simulink model "EMB_Lost_full"  (R2022a)
settings: Solver=VariableStepAuto  StartTime=0.0  StopTime=2  RelTol=1e-3
libraries: slpidlib x24, spsDCVoltageSourceLib x4, spsPermanentMagnetSynchronousMachineLib x4, spsSVPWMGenerator2LevelLib x4, spsUniversalBridgeLib x4, spsdq0toAlphaBetaZeroLib x4, spspowerguiLib x4
(part 3 of 3)

== system EMB_Lost_full/EMB_Frr/Ud_PI ==
  Ud_Target : Inport
  Ud_Actual : Inport  Port=2
  PID Controller : slpidlib/PID Controller  Controller=PI  Form=Parallel  TimeDomain=Continuous-time  UseExternalTs=off  SampleTime=-1  IntegratorMethod=Forward Euler  FilterMethod=Forward Euler  ControllerParametersSource=internal  P=0.12  I=0  UseKiTs=off  D=0.01  N=5  UseFilter=on  TunerSelectOption=Transfer Function Based (PID Tuner App)  InitialConditionSource=internal  InitialConditionForIntegrator=0  InitialConditionForFilter=0  DifferentiatorICPrevScaledInput=0  ExternalReset=none  TrackingMode=off  Kt=1  LimitOutput=on  SatLimitsSource=internal  UpperSaturationLimit=24  LowerSaturationLimit=-24  LinearizeAsGain=on  AntiWindupMode=none  Kb=1  POutMin=[]  POutMax=[]  IOutMin=[]  IOutMax=[]  DOutMin=[]  DOutMax=[]  NOutMin=[]  NOutMax=[]  SumOutMin=[]  SumOutMax=[]  SaturationOutMin=[]  SaturationOutMax=[]  PParamMin=[]  PParamMax=[]  IParamMin=[]  IParamMax=[]  DParamMin=[]  DParamMax=[]  NParamMin=[]  NParamMax=[]  KbParamMin=[]  KbParamMax=[]  KtParamMin=[]  KtParamMax=[]  KbOutMin=[]  KbOutMax=[]  KtOutMin=[]  KtOutMax=[]  IntegratorOutMin=[]  IntegratorOutMax=[]  FilterOutMin=[]  FilterOutMax=[]  SumI1OutMin=[]  SumI1OutMax=[]  SumI2OutMin=[]  SumI2OutMax=[]  SumI3OutMin=[]  SumI3OutMax=[]  SumI4OutMin=[]  SumI4OutMax=[]  SumDOutMin=[]  SumDOutMax=[]  DifferentiatorOutMin=[]  DifferentiatorOutMax=[]  FilterDiffOutCoefMin=[]  FilterDiffOutCoefMax=[]  ReciprocalOutMin=[]  ReciprocalOutMax=[]  SumDenOutMin=[]  SumDenOutMax=[]  SumNumOutMin=[]  SumNumOutMax=[]  DivideOutMin=[]  DivideOutMax=[]  UdiffTsProdOutMin=[]  UdiffTsProdOutMax=[]  NTsProdOutMin=[]  NTsProdOutMax=[]  UintegralTsProdOutMin=[]  UintegralTsProdOutMax=[]  UngainTsProdOutMin=[]  UngainTsProdOutMax=[]  IntegratorContinuousStateAttributes=''  IntegratorStateMustResolveToSignalObject=off  IntegratorRTWStateStorageClass=Auto  FilterContinuousStateAttributes=''  FilterStateMustResolveToSignalObject=off  FilterRTWStateStorageClass=Auto  ParallelPVariant=InternalParameters  IdealPVariant=Disabled  IVariant=InternalParameters  DVariant=Disabled  IntegratorVariant=Continuous  SatVariant=Enabled  AWVariant=Passthrough  PCopyVariant=Disabled  TRVariant=Disabled  FdbkBlocksVariant=Forward  IdealPFdbkVariant=Disabled  SatFdbkVariant=Disabled  DerivativeFilterVariant=Disabled  NVariant=Disabled  NCopyVariant=Disabled_SignalSpec  FilterICVariant=Disabled  IntegratorICVariant=InternalICs  ExternalResetVariant=Disabled  TRSumVariant=Passthrough  SumFdbkVariant=Disabled  SumVariant=Sum_PI  TsampFilterVariant=InternalTs  TsampNgainVariant=Passthrough  TsampIntegralVariant=Passthrough  ExternalSaturationOutDataTypeStr=Inherit: Same as second input  aMode=0
  Sum : Sum  Inputs=|+-
  Ud : Outport
  wires:
  Sum/1 -> PID Controller/1
  Ud_Actual/1 -> Sum/2
  Ud_Target/1 -> Sum/1
  PID Controller/1 -> Ud/1

== system EMB_Lost_full/EMB_Frr/Uq_PI ==
  Uq_Target : Inport
  Uq_Actual : Inport  Port=2
  PID Controller : slpidlib/PID Controller  Controller=PI  Form=Parallel  TimeDomain=Continuous-time  UseExternalTs=off  SampleTime=-1  IntegratorMethod=Forward Euler  FilterMethod=Forward Euler  ControllerParametersSource=internal  P=0.12  I=0  UseKiTs=off  D=0.01  N=5  UseFilter=on  TunerSelectOption=Transfer Function Based (PID Tuner App)  InitialConditionSource=internal  InitialConditionForIntegrator=0  InitialConditionForFilter=0  DifferentiatorICPrevScaledInput=0  ExternalReset=none  TrackingMode=off  Kt=1  LimitOutput=on  SatLimitsSource=internal  UpperSaturationLimit=24  LowerSaturationLimit=-24  LinearizeAsGain=on  AntiWindupMode=none  Kb=1  POutMin=[]  POutMax=[]  IOutMin=[]  IOutMax=[]  DOutMin=[]  DOutMax=[]  NOutMin=[]  NOutMax=[]  SumOutMin=[]  SumOutMax=[]  SaturationOutMin=[]  SaturationOutMax=[]  PParamMin=[]  PParamMax=[]  IParamMin=[]  IParamMax=[]  DParamMin=[]  DParamMax=[]  NParamMin=[]  NParamMax=[]  KbParamMin=[]  KbParamMax=[]  KtParamMin=[]  KtParamMax=[]  KbOutMin=[]  KbOutMax=[]  KtOutMin=[]  KtOutMax=[]  IntegratorOutMin=[]  IntegratorOutMax=[]  FilterOutMin=[]  FilterOutMax=[]  SumI1OutMin=[]  SumI1OutMax=[]  SumI2OutMin=[]  SumI2OutMax=[]  SumI3OutMin=[]  SumI3OutMax=[]  SumI4OutMin=[]  SumI4OutMax=[]  SumDOutMin=[]  SumDOutMax=[]  DifferentiatorOutMin=[]  DifferentiatorOutMax=[]  FilterDiffOutCoefMin=[]  FilterDiffOutCoefMax=[]  ReciprocalOutMin=[]  ReciprocalOutMax=[]  SumDenOutMin=[]  SumDenOutMax=[]  SumNumOutMin=[]  SumNumOutMax=[]  DivideOutMin=[]  DivideOutMax=[]  UdiffTsProdOutMin=[]  UdiffTsProdOutMax=[]  NTsProdOutMin=[]  NTsProdOutMax=[]  UintegralTsProdOutMin=[]  UintegralTsProdOutMax=[]  UngainTsProdOutMin=[]  UngainTsProdOutMax=[]  IntegratorContinuousStateAttributes=''  IntegratorStateMustResolveToSignalObject=off  IntegratorRTWStateStorageClass=Auto  FilterContinuousStateAttributes=''  FilterStateMustResolveToSignalObject=off  FilterRTWStateStorageClass=Auto  ParallelPVariant=InternalParameters  IdealPVariant=Disabled  IVariant=InternalParameters  DVariant=Disabled  IntegratorVariant=Continuous  SatVariant=Enabled  AWVariant=Passthrough  PCopyVariant=Disabled  TRVariant=Disabled  FdbkBlocksVariant=Forward  IdealPFdbkVariant=Disabled  SatFdbkVariant=Disabled  DerivativeFilterVariant=Disabled  NVariant=Disabled  NCopyVariant=Disabled_SignalSpec  FilterICVariant=Disabled  IntegratorICVariant=InternalICs  ExternalResetVariant=Disabled  TRSumVariant=Passthrough  SumFdbkVariant=Disabled  SumVariant=Sum_PI  TsampFilterVariant=InternalTs  TsampNgainVariant=Passthrough  TsampIntegralVariant=Passthrough  ExternalSaturationOutDataTypeStr=Inherit: Same as second input  aMode=0
  Sum : Sum  Inputs=|+-
  Uq : Outport
  wires:
  Sum/1 -> PID Controller/1
  Uq_Actual/1 -> Sum/2
  PID Controller/1 -> Uq/1
  Uq_Target/1 -> Sum/1

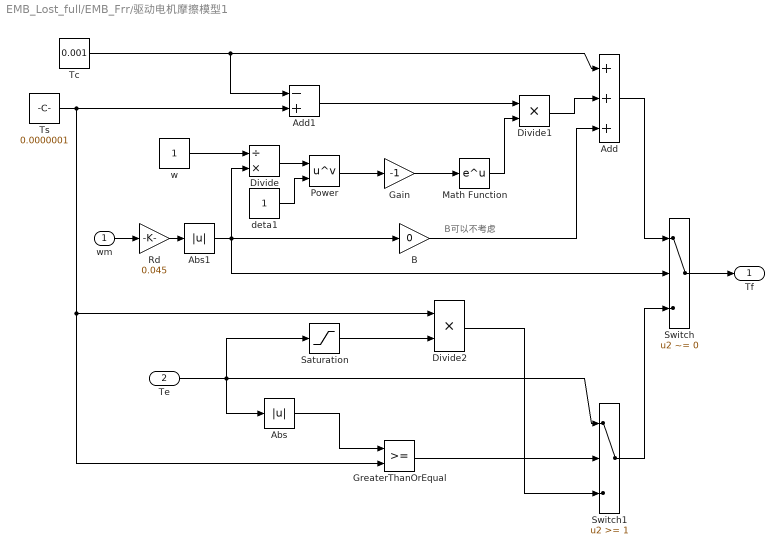
== system EMB_Lost_full/EMB_Frr/驱动电机摩擦模型1 ==
  note: B可以不考虑
  wm : Inport
  Te : Inport  Port=2
  Abs : Abs  SaturateOnIntegerOverflow=off
  Abs1 : Abs  SaturateOnIntegerOverflow=off
  Add : Sum  Inputs=+++
  Add1 : Sum  Inputs=-+
  B : Gain  Gain=0
  Divide : Product  Inputs=/*
  Divide1 : Product  Inputs=**
  Divide2 : Product  Inputs=**
  Gain : Gain  Gain=-1
  GreaterThanOrEqual : RelationalOperator  OutDataTypeStr=boolean  RndMeth=Simplest  InputSameDT=off
  Math Function : Math
  Power : Math  Operator=pow
  Rd : Gain  Gain=0.045
  Saturation : Saturate  UpperLimit=1  LowerLimit=-1
  Switch : Switch  Criteria=u2 ~= 0  SaturateOnIntegerOverflow=off  InputSameDT=off
  Switch1 : Switch  Threshold=1  SaturateOnIntegerOverflow=off  InputSameDT=off
  Tc : Constant  Value=0.001
  Ts : Constant  Value=0.0000001
  deta1 : Constant
  w : Constant
  Tf : Outport
  wires:
  Tc/1 -> Add1/1, Add/1
  Ts/1 -> Add1/2, Divide2/1, GreaterThanOrEqual/2
  B/1 -> Add/3
  w/1 -> Divide/1
  Divide/1 -> Power/1
  deta1/1 -> Power/2
  Add1/1 -> Divide1/1
  Math Function/1 -> Divide1/2
  Divide1/1 -> Add/2
  Power/1 -> Gain/1
  Gain/1 -> Math Function/1
  Switch/1 -> Tf/1
  Add/1 -> Switch/1
  Switch1/1 -> Switch/3
  Te/1 -> Saturation/1, Switch1/1, Abs/1
  Abs/1 -> GreaterThanOrEqual/1
  GreaterThanOrEqual/1 -> Switch1/2
  Saturation/1 -> Divide2/2
  Divide2/1 -> Switch1/3
  wm/1 -> Rd/1
  Rd/1 -> Abs1/1
  Abs1/1 -> Switch/2, B/1, Divide/2

== matlab function EMB_Lost_full/EMB_Ffr/EMB执行机构1/MATLAB Function ==
  data: u input; FN output; TL output
function [FN,TL] = fcn(u)
L=5; %滚动丝杠导程，mm
ip=16;%行星齿轮减速器减速比
eta_s=0.92;%滚动丝杠传动效率
eta_p=0.96; %行星齿轮传动器传动效率
s=u-0.25;
Fn=0;

if s>0.3
    Fn = -1917.2*s^3+29010.8*s^2-10197.1*s+572.4;
    if Fn<53.12
        Fn=53.12;
    end
end
if s>0 && s<=0.3
    Fn = 295.1*s;
end
if s<0
    Fn = 0;
end
if Fn>=30000
    Fn=30000;
end
Tl = 0.001*Fn/((2*pi/L)*ip*eta_s*eta_p);
FN=Fn;
TL=Tl;

== matlab function EMB_Lost_full/EMB_Ffl/EMB执行机构1/MATLAB Function ==
  data: u input; FN output; TL output
function [FN,TL] = fcn(u)
L=5; %滚动丝杠导程，mm
ip=16;%行星齿轮减速器减速比
eta_s=0.92;%滚动丝杠传动效率
eta_p=0.96; %行星齿轮传动器传动效率
s=u-0.25;
Fn=0;

if s>0.3
    Fn = -1917.2*s^3+29010.8*s^2-10197.1*s+572.4;
    if Fn<53.12
        Fn=53.12;
    end
end
if s>0 && s<=0.3
    Fn = 295.1*s;
end
if s<0
    Fn = 0;
end
if Fn>=30000
    Fn=30000;
end
Tl = 0.001*Fn/((2*pi/L)*ip*eta_s*eta_p);
FN=Fn;
TL=Tl;

== matlab function EMB_Lost_full/EMB_Ffr/EMB执行策略判断2/MATLAB Function ==
  data: Fn_Target input; y output; Fn_Actual input; Fn_Threshold input
function y = fcn(Fn_Target,Fn_Actual,Fn_Threshold)
sign=0;

if Fn_Target>0 && Fn_Actual<Fn_Threshold
    sign=2;
end

if Fn_Target>=0 && Fn_Actual>Fn_Threshold
    sign=1;
end

if Fn_Target==0 && Fn_Actual<Fn_Threshold
    sign=3;
end
y=sign;

== matlab function EMB_Lost_full/EMB_Ffl/EMB执行策略判断2/MATLAB Function ==
  data: Fn_Target input; y output; Fn_Actual input; Fn_Threshold input
function y = fcn(Fn_Target,Fn_Actual,Fn_Threshold)
sign=0;

if Fn_Target>0 && Fn_Actual<Fn_Threshold
    sign=2;
end

if Fn_Target>=0 && Fn_Actual>Fn_Threshold
    sign=1;
end

if Fn_Target==0 && Fn_Actual<Fn_Threshold
    sign=3;
end
y=sign;

== matlab function EMB_Lost_full/EMB_Frl/EMB执行机构1/MATLAB Function ==
  data: u input; FN output; TL output
function [FN,TL] = fcn(u)
L=5; %滚动丝杠导程，mm
ip=16;%行星齿轮减速器减速比
eta_s=0.92;%滚动丝杠传动效率
eta_p=0.96; %行星齿轮传动器传动效率
s=u-0.25;
Fn=0;

if s>0.3
    Fn = -1917.2*s^3+29010.8*s^2-10197.1*s+572.4;
    if Fn<53.12
        Fn=53.12;
    end
end
if s>0 && s<=0.3
    Fn = 295.1*s;
end
if s<0
    Fn = 0;
end
if Fn>=30000
    Fn=30000;
end
Tl = 0.001*Fn/((2*pi/L)*ip*eta_s*eta_p);
FN=Fn;
TL=Tl;

== matlab function EMB_Lost_full/EMB_Frl/EMB执行策略判断2/MATLAB Function ==
  data: Fn_Target input; y output; Fn_Actual input; Fn_Threshold input
function y = fcn(Fn_Target,Fn_Actual,Fn_Threshold)
sign=0;

if Fn_Target>0 && Fn_Actual<Fn_Threshold
    sign=2;
end

if Fn_Target>=0 && Fn_Actual>Fn_Threshold
    sign=1;
end

if Fn_Target==0 && Fn_Actual<Fn_Threshold
    sign=3;
end
y=sign;

== matlab function EMB_Lost_full/EMB_Frr/EMB执行机构1/MATLAB Function ==
  data: u input; FN output; TL output
function [FN,TL] = fcn(u)
L=5; %滚动丝杠导程，mm
ip=16;%行星齿轮减速器减速比
eta_s=0.92;%滚动丝杠传动效率
eta_p=0.96; %行星齿轮传动器传动效率
s=u-0.25;
Fn=0;

if s>0.3
    Fn = -1917.2*s^3+29010.8*s^2-10197.1*s+572.4;
    if Fn<53.12
        Fn=53.12;
    end
end
if s>0 && s<=0.3
    Fn = 295.1*s;
end
if s<0
    Fn = 0;
end
if Fn>=30000
    Fn=30000;
end
Tl = 0.001*Fn/((2*pi/L)*ip*eta_s*eta_p);
FN=Fn;
TL=Tl;

== matlab function EMB_Lost_full/EMB_Frr/EMB执行策略判断2/MATLAB Function ==
  data: Fn_Target input; y output; Fn_Actual input; Fn_Threshold input
function y = fcn(Fn_Target,Fn_Actual,Fn_Threshold)
sign=0;

if Fn_Target>0 && Fn_Actual<Fn_Threshold
    sign=2;
end

if Fn_Target>=0 && Fn_Actual>Fn_Threshold
    sign=1;
end

if Fn_Target==0 && Fn_Actual<Fn_Threshold
    sign=3;
end
y=sign;

== matlab function EMB_Lost_full/EMB_Self-inspection/MATLAB Function ==
  data: Total_Fn input; Fn_Target output; lost input
function Fn_Target  = fcn(Total_Fn,lost)
m=1820;
g=9.8;
a=1.27;
b=1.42;
h=0.55;
Fnmax=6500;
Zx=Total_Fn/(m*g);
Beta_fr=(b+Zx*h)/(a-Zx*h);

Ffl_Target=0.5*Zx*m*g*Beta_fr/(1+Beta_fr);
Ffr_Target=Ffl_Target;
Frl_Target=0.5*Zx*m*g*(1-Beta_fr/(1+Beta_fr));
Frr_Target=Frl_Target;
if Ffr_Target>=Fnmax || Ffl_Target>=Fnmax
    Ffr_Target=Fnmax;
    Ffl_Target=Fnmax;
    Frl_Target=0.5*(Total_Fn-2*Fnmax);
    Frr_Target=0.5*(Total_Fn-2*Fnmax);
end
Fn_Target=[Ffl_Target,Ffr_Target,Frl_Target,Frr_Target];

if lost>=1
    switch lost
        case 1
        if Fn_Target(1)+Fn_Target(3)<=Fnmax
            Fn_Target(3)=Fn_Target(1)+Fn_Target(3);
        end
        if Fn_Target(1)+Fn_Target(3)>Fnmax && Total_Fn-Fn_Target(4)<=2*Fnmax
            Fn_Target(3)=Fnmax;
            Fn_Target(2)=Total_Fn-Fn_Target(4)-Fnmax;
        end
        if Total_Fn-Fn_Target(4)>2*Fnmax && Total_Fn<=3*Fnmax
            Fn_Target(3)=Fnmax;
            Fn_Target(2)=Fnmax;
            Fn_Target(4)=Total_Fn-2*Fnmax;
        end
        if Total_Fn>3*Fnmax
            Fn_Target(2)=Fnmax;
            Fn_Target(3)=Fnmax;
            Fn_Target(4)=Fnmax;
        end
    
        case 2
        if Fn_Target(2)+Fn_Target(4)<=Fnmax
            Fn_Target(4)=Fn_Target(2)+Fn_Target(4);
        end
        if Fn_Target(2)+Fn_Target(4)>Fnmax && Total_Fn-Fn_Target(3)<=2*Fnmax
            Fn_Target(4)=Fnmax;
            Fn_Target(1)=Total_Fn-Fn_Target(3)-Fnmax;
        end
        if Total_Fn-Fn_Target(3)>2*Fnmax && Total_Fn<=3*Fnmax
            Fn_Target(4)=Fnmax;
            Fn_Target(1)=Fnmax;
            Fn_Target(3)=Total_Fn-2*Fnmax;
        end
        if Total_Fn>3*Fnmax
            Fn_Target(4)=Fnmax;
            Fn_Target(1)=Fnmax;
            Fn_Target(3)=Fnmax;
        end
    
        case 3
        if Fn_Target(1)+Fn_Target(3)<=Fnmax
            Fn_Target(1)=Fn_Target(1)+Fn_Target(3);
        end
        if Fn_Target(1)+Fn_Target(3)>Fnmax && Total_Fn-Fn_Target(4)<=2*Fnmax
            Fn_Target(1)=Fnmax;
            Fn_Target(2)=Total_Fn-Fn_Target(4)-Fnmax;
        end
        if Total_Fn-Fn_Target(4)>2*Fnmax && Total_Fn<=3*Fnmax
            Fn_Target(1)=Fnmax;
            Fn_Target(2)=Fnmax;
            Fn_Target(4)=Total_Fn-2*Fnmax;
        end
        if Total_Fn>3*Fnmax
            Fn_Target(1)=Fnmax;
            Fn_Target(2)=Fnmax;
            Fn_Target(4)=Fnmax;
        end
    
        case 4
        if Fn_Target(2)+Fn_Target(4)<=Fnmax
            Fn_Target(2)=Fn_Target(2)+Fn_Target(4);
        end
        if Fn_Target(2)+Fn_Target(4)>Fnmax && Total_Fn-Fn_Target(3)<=2*Fnmax
            Fn_Target(2)=Fnmax;
            Fn_Target(1)=Total_Fn-Fn_Target(3)-Fnmax;
        end
        if Total_Fn-Fn_Target(3)>2*Fnmax && Total_Fn<=3*Fnmax
            Fn_Target(2)=Fnmax;
            Fn_Target(1)=Fnmax;
            Fn_Target(3)=Total_Fn-2*Fnmax;
        end
        if Total_Fn>3*Fnmax
            Fn_Target(2)=Fnmax;
            Fn_Target(1)=Fnmax;
            Fn_Target(3)=Fnmax;
        end
    end
end
